simulink model "dualConversionSuperheterodyneCBandReceiver"  (R2021b)
settings: Solver=VariableStepAuto  StartTime=0.0  StopTime=10.0  RelTol=1e-3
undefined symbols (not defined in the file): fdesignblkfcn, gcbh
libraries: dsparch4 x6, dspsrcs4 x4
settings Model: Creator=Zireael  LastModifiedBy=Zireael

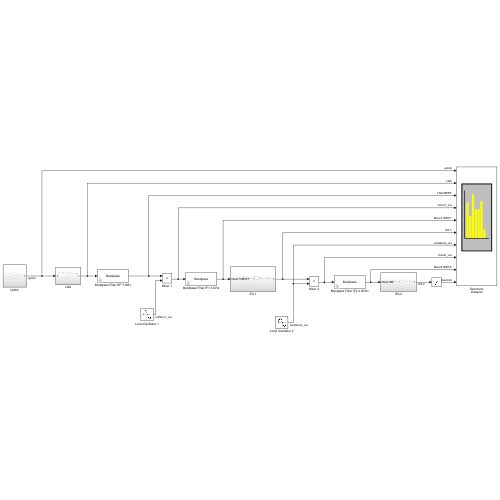
[thumbnail: Simulink's stored preview of the top-level diagram]
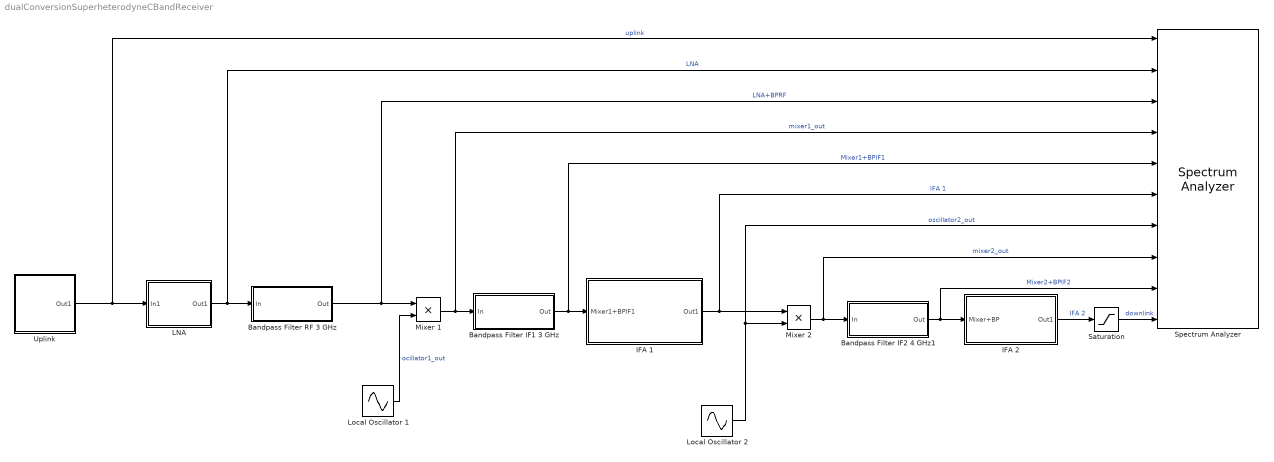
== system dualConversionSuperheterodyneCBandReceiver ==
  Bandpass Filter IF1 3 GHz : Subsystem  DialogController=fdesignblkfcn  InitFcn=fdesignblkfcn(gcbh, {'InitFcn'});  mask(Bandpass Filter){}
      mask help: Design a bandpass filter
      settings: CopyFcn=fdesignblkfcn(gcbh, {'CopyFcn'});
      mask Help: helpview(mapfilelocation('dsp'), 'dspbandpassfilter');
      mask Display: disp('Bandpass');
  Bandpass Filter IF2 4 GHz1 : Subsystem  DialogController=fdesignblkfcn  InitFcn=fdesignblkfcn(gcbh, {'InitFcn'});  mask(Bandpass Filter){}
      mask help: Design a bandpass filter
      settings: CopyFcn=fdesignblkfcn(gcbh, {'CopyFcn'});
      mask Help: helpview(mapfilelocation('dsp'), 'dspbandpassfilter');
      mask Display: disp('Bandpass');
  Bandpass Filter RF 3 GHz : Subsystem  DialogController=fdesignblkfcn  InitFcn=fdesignblkfcn(gcbh, {'InitFcn'});  mask(Bandpass Filter){}
      mask help: Design a bandpass filter
      settings: CopyFcn=fdesignblkfcn(gcbh, {'CopyFcn'});
      mask Help: helpview(mapfilelocation('dsp'), 'dspbandpassfilter');
      mask Display: disp('Bandpass');
  IFA 1 : Subsystem
  IFA 2 : Subsystem
  LNA : Subsystem
  Local Oscillator 1 : Sin  Frequency=2*pi*2225e6  SampleTime=1/(50e9)
  Local Oscillator 2 : Sin  Frequency=2*pi*2225e6  SampleTime=1/(50e9)
  Mixer 1 : Product
  Mixer 2 : Product
  Saturation : Saturate  UpperLimit=0.9e4  LowerLimit=-0.9e4
  Spectrum Analyzer : SpectrumAnalyzer  NumInputPorts=10
  Uplink : Subsystem
  wires:
  Local Oscillator 1/1 -> Mixer 1/2  "ocillator1_out"
  Uplink/1(Out1) -> Spectrum Analyzer/1, LNA/1(In1)  "uplink"
  Bandpass Filter RF 3 GHz/1(Out) -> Spectrum Analyzer/3, Mixer 1/1  "LNA+BPRF"
  LNA/1(Out1) -> Spectrum Analyzer/2, Bandpass Filter RF 3 GHz/1(In)  "LNA"
  Mixer 1/1 -> Spectrum Analyzer/4, Bandpass Filter IF1 3 GHz/1(In)  "mixer1_out"
  Bandpass Filter IF1 3 GHz/1(Out) -> Spectrum Analyzer/5, IFA 1/1(Mixer1+BPIF1)  "Mixer1+BPIF1"
  Local Oscillator 2/1 -> Spectrum Analyzer/7, Mixer 2/2  "oscillator2_out"
  Mixer 2/1 -> Spectrum Analyzer/8, Bandpass Filter IF2 4 GHz1/1(In)  "mixer2_out"
  Bandpass Filter IF2 4 GHz1/1(Out) -> Spectrum Analyzer/9, IFA 2/1(Mixer+BP)  "Mixer2+BPIF2"
  IFA 1/1(Out1) -> Spectrum Analyzer/6, Mixer 2/1  "IFA 1"
  IFA 2/1(Out1) -> Saturation/1  "IFA 2"
  Saturation/1 -> Spectrum Analyzer/10  "downlink"

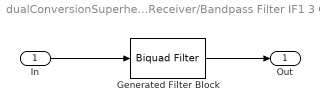
== system dualConversionSuperheterodyneCBandReceiver/Bandpass Filter IF1 3 GHz ==
  In : Inport
  Generated Filter Block : dsparch4/Biquad Filter  Tag=BlockMethodSubSystem  FilterSource=Dialog parameters  CoeffSource=Specify via dialog  FilterObject=BQF  IIRFiltStruct=Direct form II  BiQuadCoeffs=[0.045800424595222218 0 -0.045800424595222218 1 -1.49237351358389714 0.993808592132404689;0.015329352312781765 0 -0.015329352312781765 1 -1.43131811463111913 0.993502217044615277;0.0103606247840062719 0 -0.0103606247840062719 1 -1.46745730699721344 0.991192023750536499;0.0146167790338295311 0 -0.0146167790338295311 1 -1.45394760309045812 0.99109749167996064;0.0648446569067554351 0 -0.0648446569067554351 1 -1.50738927731367967 0.998641094086305525;0.00936076343834263414 0 -0.00936076343834263414 1 -1.42213817852353408 0.99854604518880985;0.0228861499994813498 0 -0.0228861499994813498 1 -1.48067266509199102 0.992133374334369544;0.0124518110188895064 0 -0.0124518110188895064 1 -1.4414682482231207 0.991885766532117352;0.0610038980140942058 0 -0.0610038980140942058 1 -1.50153636770328802 0.996047228844719967;0.757595368550774695 0 -0.757595368550774695 1 -1.42461460731617251 0.995798956657499179]  ScaleValues=[0.00411230562279772324;1;1;1;1;1;1;1;1;1;1]  IC=0  ICnum=0  ICden=0  a0Flag=Warning  optimizeScaleValues=off  ScaleValueMode=Specify via input port (g)  InputProcessing=Columns as channels (frame based)  roundingMode=Floor  overflowMode=off  scaleValueFracLength=14  denProdOutputFracLength=30  denAccumFracLength=30  secondMemoryFracLength=15
  Out : Outport  VectorParamsAs1DForOutWhenUnconnected=off
  wires:
  In/1 -> Generated Filter Block/1
  Generated Filter Block/1 -> Out/1

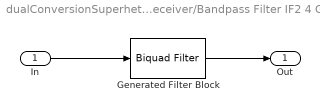
== system dualConversionSuperheterodyneCBandReceiver/Bandpass Filter IF2 4 GHz1 ==
  In : Inport
  Generated Filter Block : dsparch4/Biquad Filter  Tag=BlockMethodSubSystem  FilterSource=Dialog parameters  CoeffSource=Specify via dialog  FilterObject=BQF  IIRFiltStruct=Direct form II  BiQuadCoeffs=[0.045800424595222218 0 -0.045800424595222218 1 -1.49237351358389714 0.993808592132404689;0.015329352312781765 0 -0.015329352312781765 1 -1.43131811463111913 0.993502217044615277;0.0103606247840062719 0 -0.0103606247840062719 1 -1.46745730699721344 0.991192023750536499;0.0146167790338295311 0 -0.0146167790338295311 1 -1.45394760309045812 0.99109749167996064;0.0648446569067554351 0 -0.0648446569067554351 1 -1.50738927731367967 0.998641094086305525;0.00936076343834263414 0 -0.00936076343834263414 1 -1.42213817852353408 0.99854604518880985;0.0228861499994813498 0 -0.0228861499994813498 1 -1.48067266509199102 0.992133374334369544;0.0124518110188895064 0 -0.0124518110188895064 1 -1.4414682482231207 0.991885766532117352;0.0610038980140942058 0 -0.0610038980140942058 1 -1.50153636770328802 0.996047228844719967;0.757595368550774695 0 -0.757595368550774695 1 -1.42461460731617251 0.995798956657499179]  ScaleValues=[0.00411230562279772324;1;1;1;1;1;1;1;1;1;1]  IC=0  ICnum=0  ICden=0  a0Flag=Warning  optimizeScaleValues=off  ScaleValueMode=Specify via input port (g)  InputProcessing=Columns as channels (frame based)  roundingMode=Floor  overflowMode=off  scaleValueFracLength=14  denProdOutputFracLength=30  denAccumFracLength=30  secondMemoryFracLength=15
  Out : Outport  VectorParamsAs1DForOutWhenUnconnected=off
  wires:
  In/1 -> Generated Filter Block/1
  Generated Filter Block/1 -> Out/1

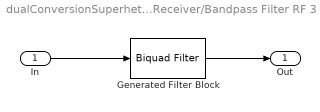
== system dualConversionSuperheterodyneCBandReceiver/Bandpass Filter RF 3 GHz ==
  In : Inport
  Generated Filter Block : dsparch4/Biquad Filter  Tag=BlockMethodSubSystem  FilterSource=Dialog parameters  CoeffSource=Specify via dialog  FilterObject=BQF  IIRFiltStruct=Direct form II  BiQuadCoeffs=[0.0458057266197743618 0 -0.0458057266197743618 1 -1.45437320283285776 0.993800154047264295;0.01531173562674705 0 -0.01531173562674705 1 -1.39150376301706036 0.993510652600055;0.0103561680167830183 0 -0.0103561680167830183 1 -1.42878022084028666 0.991189419085551582;0.0146134254621030774 0 -0.0146134254621030774 1 -1.41487088836209862 0.991100096103380457;0.0646086918377938857 0 -0.0646086918377938857 1 -1.4696829304609409 0.998638477918037726;0.00941269145149956944 0 -0.00941269145149956944 1 -1.38187454124205944 0.998548661114929459;0.0228497542345437281 0 -0.0228497542345437281 1 -1.44236668000108015 0.992126552789106553;0.012674652641078003 0 -0.012674652641078003 1 -1.4020008435493605 0.991892586421807332;0.0599553530961037806 0 -0.0599553530961037806 1 -1.46374389621031886 0.996040393415140501;0.735069498699384982 0 -0.735069498699384982 1 -1.38452696041598822 0.995805790430190463]  ScaleValues=[0.00424255902808068006;1;1;1;1;1;1;1;1;1;1]  IC=0  ICnum=0  ICden=0  a0Flag=Warning  optimizeScaleValues=off  ScaleValueMode=Specify via input port (g)  InputProcessing=Columns as channels (frame based)  roundingMode=Floor  overflowMode=off  scaleValueFracLength=14  denProdOutputFracLength=30  denAccumFracLength=30  secondMemoryFracLength=15
  Out : Outport  VectorParamsAs1DForOutWhenUnconnected=off
  wires:
  In/1 -> Generated Filter Block/1
  Generated Filter Block/1 -> Out/1

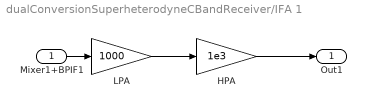
== system dualConversionSuperheterodyneCBandReceiver/IFA 1 ==
  Mixer1+BPIF1 : Inport
  HPA : Gain  Gain=1e3
  LPA : Gain  Gain=1000
  Out1 : Outport
  wires:
  Mixer1+BPIF1/1 -> LPA/1
  LPA/1 -> HPA/1
  HPA/1 -> Out1/1

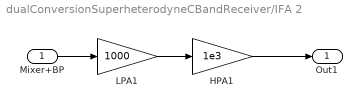
== system dualConversionSuperheterodyneCBandReceiver/IFA 2 ==
  Mixer+BP : Inport
  HPA1 : Gain  Gain=1e3
  LPA1 : Gain  Gain=1000
  Out1 : Outport
  wires:
  LPA1/1 -> HPA1/1
  HPA1/1 -> Out1/1
  Mixer+BP/1 -> LPA1/1

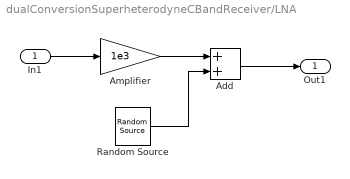
== system dualConversionSuperheterodyneCBandReceiver/LNA ==
  In1 : Inport
  Add : Sum
  Amplifier : Gain  Gain=1e3
  Random Source : dspsrcs4/Random Source  SrcType=Gaussian  NormMethod=Ziggurat  CltLength=12  MinVal=0  MaxVal=1  MeanVal=0  VarVal=1e-3  RepMode=Not repeatable  rawSeed=1  IsInherit=off  SampMode=Discrete  SampTime=1/(50e9)  SampFrame=1  DataType=Double  OutComplex=Real  OutputFrames=off
  Out1 : Outport
  wires:
  Random Source/1 -> Add/2
  Amplifier/1 -> Add/1
  Add/1 -> Out1/1
  In1/1 -> Amplifier/1

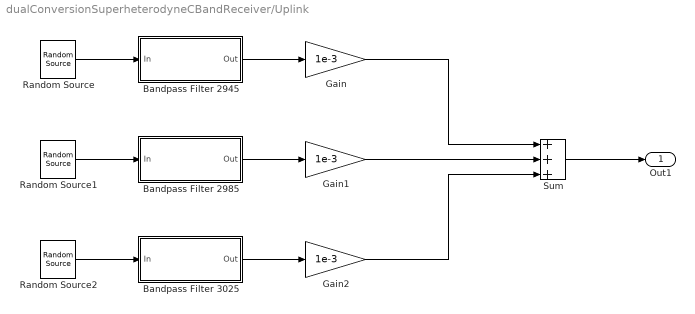
== system dualConversionSuperheterodyneCBandReceiver/Uplink ==
  Bandpass Filter 2945 : Subsystem  DialogController=fdesignblkfcn  InitFcn=fdesignblkfcn(gcbh, {'InitFcn'});  mask(Bandpass Filter){}
      mask help: Design a bandpass filter
      settings: CopyFcn=fdesignblkfcn(gcbh, {'CopyFcn'});
      mask Help: helpview(mapfilelocation('dsp'), 'dspbandpassfilter');
      mask Display: disp('Bandpass');
  Bandpass Filter 2985 : Subsystem  DialogController=fdesignblkfcn  InitFcn=fdesignblkfcn(gcbh, {'InitFcn'});  mask(Bandpass Filter){}
      mask help: Design a bandpass filter
      settings: CopyFcn=fdesignblkfcn(gcbh, {'CopyFcn'});
      mask Help: helpview(mapfilelocation('dsp'), 'dspbandpassfilter');
      mask Display: disp('Bandpass');
  Bandpass Filter 3025 : Subsystem  DialogController=fdesignblkfcn  InitFcn=fdesignblkfcn(gcbh, {'InitFcn'});  mask(Bandpass Filter){}
      mask help: Design a bandpass filter
      settings: CopyFcn=fdesignblkfcn(gcbh, {'CopyFcn'});
      mask Help: helpview(mapfilelocation('dsp'), 'dspbandpassfilter');
      mask Display: disp('Bandpass');
  Gain : Gain  Gain=1e-3
  Gain1 : Gain  Gain=1e-3
  Gain2 : Gain  Gain=1e-3
  Random Source : dspsrcs4/Random Source  SrcType=Gaussian  NormMethod=Ziggurat  CltLength=12  MinVal=0  MaxVal=1  MeanVal=0  VarVal=1  RepMode=Not repeatable  rawSeed=1  IsInherit=off  SampMode=Discrete  SampTime=1/(50e9)  SampFrame=1  DataType=Double  OutComplex=Real  OutputFrames=off
  Random Source1 : dspsrcs4/Random Source  SrcType=Gaussian  NormMethod=Ziggurat  CltLength=12  MinVal=0  MaxVal=1  MeanVal=0  VarVal=1  RepMode=Not repeatable  rawSeed=1  IsInherit=off  SampMode=Discrete  SampTime=1/(50e9)  SampFrame=1  DataType=Double  OutComplex=Real  OutputFrames=off
  Random Source2 : dspsrcs4/Random Source  SrcType=Gaussian  NormMethod=Ziggurat  CltLength=12  MinVal=0  MaxVal=1  MeanVal=0  VarVal=1  RepMode=Not repeatable  rawSeed=1  IsInherit=off  SampMode=Discrete  SampTime=1/(50e9)  SampFrame=1  DataType=Double  OutComplex=Real  OutputFrames=off
  Sum : Sum  Inputs=+++
  Out1 : Outport
  wires:
  Random Source/1 -> Bandpass Filter 2945/1(In)
  Bandpass Filter 2945/1(Out) -> Gain/1
  Bandpass Filter 2985/1(Out) -> Gain1/1
  Random Source1/1 -> Bandpass Filter 2985/1(In)
  Random Source2/1 -> Bandpass Filter 3025/1(In)
  Bandpass Filter 3025/1(Out) -> Gain2/1
  Sum/1 -> Out1/1
  Gain/1 -> Sum/1
  Gain1/1 -> Sum/2
  Gain2/1 -> Sum/3

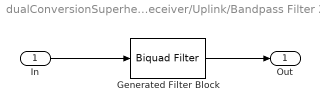
== system dualConversionSuperheterodyneCBandReceiver/Uplink/Bandpass Filter 2945 ==
  In : Inport
  Generated Filter Block : dsparch4/Biquad Filter  Tag=BlockMethodSubSystem  FilterSource=Dialog parameters  CoeffSource=Specify via dialog  FilterObject=BQF  IIRFiltStruct=Direct form II  BiQuadCoeffs=[0.00391601063166015662 0 -0.00391601063166015662 1 -1.46987896016374231 0.999784822825606101;0.00148044188753657124 0 -0.00148044188753657124 1 -1.46453048469215386 0.9997839065925469;0.00115383107801688692 0 -0.00115383107801688692 1 -1.46770084317129879 0.99957841078172649;0.00094730551194260014 0 -0.00094730551194260014 1 -1.46641678239278628 0.999577980550796719;0.00174942855977432859 0 -0.00174942855977432859 1 -1.46892509262117898 0.999651620321149736;0.000836465162084115655 0 -0.000836465162084115655 1 -1.46529495754295969 0.999650614257482806;0.00317262394377629525 0 -0.00317262394377629525 1 -1.47039902583043869 0.999955026160952332;0.000382474873925192139 0 -0.000382474873925192139 1 -1.46425705672080397 0.999954806158664833;0.00357511039278767115 0 -0.00357511039278767115 1 -1.46944751533388174 0.999711959935413286;0.00133546302840172179 0 -0.00133546302840172179 1 -1.46485790912283642 0.99971090783189942;0.000643959473675208369 0 -0.000643959473675208369 1 -1.46705222777919109 0.999568774242084457;0.00138556699835995045 0 -0.00138556699835995045 1 -1.46833432074380066 0.999606441706998528;0.00114221336578256786 0 -0.00114221336578256786 1 -1.46582232447542915 0.999605655614189459;0.00409147471494122634 0 -0.00409147471494122634 1 -1.47020076696388413 0.999867035634280921;0.734309306340847567 0 -0.734309306340847567 1 -1.46432718863438827 0.999866413723099479]  ScaleValues=[0.000151073531716674537;1;1;1;1;1;1;1;1;1;1;1;1;1;1;1]  IC=0  ICnum=0  ICden=0  a0Flag=Warning  optimizeScaleValues=off  ScaleValueMode=Specify via input port (g)  InputProcessing=Columns as channels (frame based)  roundingMode=Floor  overflowMode=off  scaleValueFracLength=14  denProdOutputFracLength=30  denAccumFracLength=30  secondMemoryFracLength=15
  Out : Outport  VectorParamsAs1DForOutWhenUnconnected=off
  wires:
  In/1 -> Generated Filter Block/1
  Generated Filter Block/1 -> Out/1

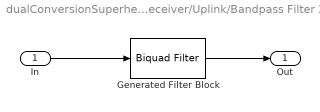
== system dualConversionSuperheterodyneCBandReceiver/Uplink/Bandpass Filter 2985 ==
  In : Inport
  Generated Filter Block : dsparch4/Biquad Filter  Tag=BlockMethodSubSystem  FilterSource=Dialog parameters  CoeffSource=Specify via dialog  FilterObject=BQF  IIRFiltStruct=Direct form II  BiQuadCoeffs=[0.0039571986993747069 0 -0.0039571986993747069 1 -1.46304466882617024 0.999784818230979644;0.00152121618225881387 0 -0.00152121618225881387 1 -1.45766724604227771 0.999783911187176466;0.00113362100656203696 0 -0.00113362100656203696 1 -1.46085623258113184 0.999578408625500847;0.00090696106066402867 0 -0.00090696106066402867 1 -1.45956522517878584 0.999577982707027357;0.00179040985118408867 0 -0.00179040985118408867 1 -1.46208659048957657 0.99965161527625368;0.000829779491448935039 0 -0.000829779491448935039 1 -1.45843681376259582 0.999650619302370869;0.00277113352129717107 0 -0.00277113352129717107 1 -1.46356631222902234 0.999955025057876146;0.000479552455573597569 0 -0.000479552455573597569 1 -1.45739108905466019 0.999954807261747347;0.0032930249567736658 0 -0.0032930249567736658 1 -1.46261141124832861 0.99971195466022067;0.00140308185883153652 0 -0.00140308185883153652 1 -1.45799696877776874 0.999710913107093146;0.000605783626999674765 0 -0.000605783626999674765 1 -1.46020417461524166 0.999568774242084679;0.00146794003942045176 0 -0.00146794003942045176 1 -1.46149294097960669 0.999606437765956257;0.00111246400430499459 0 -0.00111246400430499459 1 -1.45896735429559765 0.999605659555225401;0.00413239450349704284 0 -0.00413239450349704284 1 -1.46336762282523902 0.999867032516346343;0.729291005500355638 0 -0.729291005500355638 1 -1.45746224958927928 0.999866416841032724]  ScaleValues=[0.00014763811494195416;1;1;1;1;1;1;1;1;1;1;1;1;1;1;1]  IC=0  ICnum=0  ICden=0  a0Flag=Warning  optimizeScaleValues=off  ScaleValueMode=Specify via input port (g)  InputProcessing=Columns as channels (frame based)  roundingMode=Floor  overflowMode=off  scaleValueFracLength=14  denProdOutputFracLength=30  denAccumFracLength=30  secondMemoryFracLength=15
  Out : Outport  VectorParamsAs1DForOutWhenUnconnected=off
  wires:
  In/1 -> Generated Filter Block/1
  Generated Filter Block/1 -> Out/1

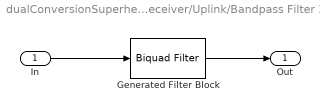
== system dualConversionSuperheterodyneCBandReceiver/Uplink/Bandpass Filter 3025 ==
  In : Inport
  Generated Filter Block : dsparch4/Biquad Filter  Tag=BlockMethodSubSystem  FilterSource=Dialog parameters  CoeffSource=Specify via dialog  FilterObject=BQF  IIRFiltStruct=Direct form II  BiQuadCoeffs=[0.0041256983846294313 0 -0.0041256983846294313 1 -1.45641434300686079 0.999876570270396225;0.000846461925651923776 0 -0.000846461925651923776 1 -1.45065837654863872 0.999876021787243108;0.00316281002746601671 0 -0.00316281002746601671 1 -1.45505795260168225 0.999724746235327588;0.000739874834793836662 0 -0.000739874834793836662 1 -1.45180264610755216 0.999724055206255402;0.00106136655701590367 0 -0.00106136655701590367 1 -1.45413102381410497 0.999685882186495567;0.000813004343158884647 0 -0.000813004343158884647 1 -1.45267659317948516 0.999685530101889763;0.00298428692621205026 0 -0.00298428692621205026 1 -1.45584450679421273 0.999790455068524375;0.000576590278815982109 0 -0.000576590278815982109 1 -1.45110699144220878 0.99978968900982701;0.00383235619244647182 0 -0.00383235619244647182 1 -1.45671227156301986 0.999974697226974851;0.000136069045136195726 0 -0.000136069045136195726 1 -1.45050130035144265 0.999974575873675997;0.00396346911404278201 0 -0.00396346911404278201 1 -1.45616053170087478 0.999831449476697109;0.00116180904810861928 0 -0.00116180904810861928 1 -1.4508483875207967 0.999830758377641571;0.00289514858526818825 0 -0.00289514858526818825 1 -1.45460662325497703 0.999701651425615623;0.000903317448437241386 0 -0.000903317448437241386 1 -1.45222239942067821 0.999701103034971617;0.000625675204039235393 0 -0.000625675204039235393 1 -1.4536428151125369 0.99967783367456875;0.00104140183326304793 0 -0.00104140183326304793 1 -1.45315399253182176 0.999677712355696135;0.00208701839296857082 0 -0.00208701839296857082 1 -1.45547396780669502 0.999754593164801753;0.00122124186804986536 0 -0.00122124186804986536 1 -1.45142773894965105 0.99975382713158667;0.00378569945395675587 0 -0.00378569945395675587 1 -1.45659976109621203 0.999924712137392313;0.728551325428745233 0 -0.728551325428745233 1 -1.45054170651787739 0.999924359972602095]  ScaleValues=[0.00013174934774159427;1;1;1;1;1;1;1;1;1;1;1;1;1;1;1;1;1;1;1;1]  IC=0  ICnum=0  ICden=0  a0Flag=Warning  optimizeScaleValues=off  ScaleValueMode=Specify via input port (g)  InputProcessing=Columns as channels (frame based)  roundingMode=Floor  overflowMode=off  scaleValueFracLength=14  denProdOutputFracLength=30  denAccumFracLength=30  secondMemoryFracLength=15
  Out : Outport  VectorParamsAs1DForOutWhenUnconnected=off
  wires:
  Generated Filter Block/1 -> Out/1
  In/1 -> Generated Filter Block/1
